simulink model "full_maneuver_platoon_new_strategy"  (R2019a)
settings: Solver=VariableStepAuto  StartTime=0.0  StopTime=70  FixedStep=0.1  MaxStep=0.05  RelTol=1e-3
libraries: simulink x97, dspsigops x7, powerlib_meascontrol x7, autolibshared x7
(part 4 of 7)

== system full_maneuver_platoon_new_strategy/p1/safeErrors ==
  errors : Inport
  AND : Logic  IconShape=distinctive  AllPortsSameDT=off  OutDataTypeStr=boolean
  Compare To Constant4 : simulink/Logic and Bit Operations/Compare To Constant  relop=>=  const=-0.1  OutDataTypeStr=boolean
  Demux : Demux  Outputs=2
  safetyFlag : Outport
  wires:
  Compare To Constant4/1 -> Demux/1
  errors/1 -> Compare To Constant4/1
  AND/1 -> safetyFlag/1
  Demux/1 -> AND/1
  Demux/2 -> AND/2

== system full_maneuver_platoon_new_strategy/p1/safeErrors1 ==
  errors : Inport
  AND : Logic  IconShape=distinctive  AllPortsSameDT=off  OutDataTypeStr=boolean
  Compare To Constant4 : simulink/Logic and Bit Operations/Compare To Constant  relop=>=  const=-0.1  OutDataTypeStr=boolean
  Demux : Demux  Outputs=2
  safetyFlag : Outport
  wires:
  Demux/2 -> AND/2
  Demux/1 -> AND/1
  AND/1 -> safetyFlag/1
  errors/1 -> Compare To Constant4/1
  Compare To Constant4/1 -> Demux/1

== system full_maneuver_platoon_new_strategy/p1/safeErrors2 ==
  errors : Inport
  AND : Logic  IconShape=distinctive  AllPortsSameDT=off  OutDataTypeStr=boolean
  Compare To Constant4 : simulink/Logic and Bit Operations/Compare To Constant  relop=>=  const=-0.1  OutDataTypeStr=boolean
  Demux : Demux  Outputs=2
  safetyFlag : Outport
  wires:
  Compare To Constant4/1 -> Demux/1
  errors/1 -> Compare To Constant4/1
  AND/1 -> safetyFlag/1
  Demux/1 -> AND/1
  Demux/2 -> AND/2

== system full_maneuver_platoon_new_strategy/p1/steadyState ==
  u : Inport
  AND : Logic  IconShape=distinctive  AllPortsSameDT=off  OutDataTypeStr=boolean
  Abs2 : Abs
  Compare To Constant2 : simulink/Logic and Bit Operations/Compare To Constant  relop=<=  const=0.2  OutDataTypeStr=boolean
  Demux : Demux  Outputs=2
  Mux : Mux  Inputs=2
  Transport Delay2 : TransportDelay
  ssFlag : Outport
  wires:
  Demux/2 -> AND/2
  Mux/1 -> Abs2/1
  Compare To Constant2/1 -> Demux/1
  AND/1 -> ssFlag/1
  Transport Delay2/1 -> Mux/1
  Demux/1 -> AND/1
  Abs2/1 -> Compare To Constant2/1
  u/1 -> Mux/2, Transport Delay2/1

== system full_maneuver_platoon_new_strategy/p2/Lateral Control ==
  <Y> : Inport
  <r> : Inport  Port=2
  startLaneChange : Inport  Port=3
  yRef : Inport  Port=4
  Demux2 : Demux
  Full State Observer : Subsystem
  Gain1 : Gain  Gain=Klat  Multiplication=Matrix(K*u)
  Integrator : Integrator  InitialCondition=y0
  Mux : Mux  Inputs=2
  Pad : dspsigops/Pad  padAlong=Columns  dimsToPad=1  valSrc=Specify via dialog  padVal=0  spec=Output size  padNumOutRowsSpecMethod=User-specified  numOutRows=4  padNumOutColsSpecMethod=User-specified  numOutCols=1  isVarDimsMode=off  padBeginning=0  padEnd=0  outSizeMode=User-specified  outSize=1  padSigAt=End  trunc_flag=None  roundingMode=Floor  overflowMode=off  truncOrWrapMode=Truncate  wrap_flag=None
      settings: SourceProductName=DSP System Toolbox  SourceProductBaseCode=DS
  Rate Limiter : RateLimiter  RisingSlewLimit=maxDeltaDot  FallingSlewLimit=-maxDeltaDot  SampleTimeMode=inherited
  Saturation : Saturate  UpperLimit=maxDelta  LowerLimit=-maxDelta
  Scope : Scope  NumInputPorts=4
  Scope1 : Scope
  Sum : Sum  Inputs=|+-
  Sum2 : Sum  Inputs=|+-
  Triggered Subsystem1 : Subsystem  TreatAsAtomicUnit=on
  delta : Outport
  wires:
  Rate Limiter/1 -> Full State Observer/2(delta), Scope1/1, delta/1  "delta"
  Demux2/1 -> Scope/1
  Integrator/1 -> Sum2/2, Pad/1
  Gain1/1 -> Saturation/1
  <r>/1 -> Mux/2
  Full State Observer/1(xhat) -> Sum/2, Demux2/1  "estStates"
  Sum/1 -> Gain1/1
  Pad/1 -> Sum/1
  Mux/1 -> Full State Observer/1(measuredOutputs)
  Demux2/4 -> Scope/4
  Demux2/2 -> Scope/2
  Sum2/1 -> Integrator/1
  Saturation/1 -> Rate Limiter/1
  Demux2/3 -> Scope/3
  Triggered Subsystem1/1(Out1) -> Sum2/1
  <Y>/1 -> Mux/1
  startLaneChange/1 -> Triggered Subsystem1/Trigger
  yRef/1 -> Triggered Subsystem1/1(In1)

== system full_maneuver_platoon_new_strategy/p2/Regular Vehicle Following ==
  ego : Inport
  leader : Inport  Port=2
  extraSpaceFlag : Inport  Port=3
  Bus Selector : BusSelector  OutputSignals=X,Xdot,u
  Bus Selector1 : BusSelector  OutputSignals=X,Xdot
  Chart : Stateflow chart  BlockKeywords=__PRM__SERIALIZED__DATA__:Stateflow Chart,Stateflow Diagram  TreatAsAtomicUnit=on
  Compare To Constant : simulink/Logic and Bit Operations/Compare To Constant  relop=<  const=5*maxHeadwayError  OutDataTypeStr=boolean
  Compare To Constant1 : simulink/Logic and Bit Operations/Compare To Constant  relop=>  const=0  OutDataTypeStr=boolean
  Compute Errors : Subsystem
  Free Flow Velocity Control : Subsystem  TreatAsAtomicUnit=on
  Minimum Velocity Control : Subsystem  TreatAsAtomicUnit=on
  Mux : Mux  Inputs=2
  Rate Limiter : RateLimiter  RisingSlewLimit=maxJerk  FallingSlewLimit=minJerk  SampleTimeMode=inherited
  Rate Limiter1 : RateLimiter  RisingSlewLimit=maxComfJerk  FallingSlewLimit=minComfJerk  SampleTimeMode=inherited
  Scope2 : Scope
  Sum1 : Sum  Inputs=-+|
  Sum6 : Sum  Inputs=-+|
  Switch1 : Switch  Criteria=u2 > Threshold
  Veh Following : Subsystem  TreatAsAtomicUnit=on
  comf saturation : Saturate  UpperLimit=maxComfAccel  LowerLimit=minComfAccel
  freeFlowVel : Constant  Value=freeFlowVel
  output : Scope
  safe saturation : Saturate  UpperLimit=maxAcceleration  LowerLimit=minAcceleration
  vMin : Constant  Value=vMin
  veh foll state : Scope  NumInputPorts=2
  u : Outport
  errors : Outport  Port=2
  gap : Outport  Port=3
  leaderInRange : Outport  Port=4
  wires:
  Bus Selector/2 -> Sum1/1, Sum6/1, Compute Errors/2(vf)  "<Xdot>"
  Bus Selector/1 -> Compute Errors/1(xf)  "<X>"
  extraSpaceFlag/1 -> Compute Errors/5(extraSpaceFlag)
  Compute Errors/1(eh) -> Mux/1, Veh Following/1(eh), Compare To Constant/1
  Compare To Constant/1 -> leaderInRange/1, Chart/1(leaderWithinRange), Free Flow Velocity Control/3(intReset), Veh Following/4(intReset)
  ego/1 -> Bus Selector/1
  Compute Errors/3("gap ") -> gap/1
  Compute Errors/4(unsafeFlag) -> Chart/3(unsafeFlag), Switch1/2, Scope2/1
  Rate Limiter1/1 -> Switch1/3  "sat(u)"
  Bus Selector/3 -> Veh Following/3(realInput), Minimum Velocity Control/2(realInput), Free Flow Velocity Control/2(realInput)  "<u>"
  Chart/2(u) -> safe saturation/1, comf saturation/1, veh foll state/2
  Switch1/1 -> u/1, output/1
  Rate Limiter/1 -> Switch1/1  "sat(u)"
  safe saturation/1 -> Rate Limiter/1
  comf saturation/1 -> Rate Limiter1/1
  Compute Errors/2(ev) -> Veh Following/2(ev), Mux/2
  Free Flow Velocity Control/1(u) -> Chart/5(freeFlowVelControl)
  Bus Selector1/1 -> Compute Errors/3(xl)  "<X>"
  Mux/1 -> errors/1
  Chart/1(state) -> veh foll state/1
  leader/1 -> Bus Selector1/1
  Bus Selector1/2 -> Compute Errors/4(vl)  "<Xdot>"
  Veh Following/1(u) -> Chart/4(vehFoll)  "uVehFoll"
  Sum6/1 -> Compare To Constant1/1, Chart/2(velDiff), Minimum Velocity Control/1(ev)
  Minimum Velocity Control/1(u) -> Chart/6(minVelControl)  "minVelControl"
  vMin/1 -> Sum6/2
  freeFlowVel/1 -> Sum1/2
  Sum1/1 -> Free Flow Velocity Control/1(ev)
  Compare To Constant1/1 -> Minimum Velocity Control/3(intReset)

== system full_maneuver_platoon_new_strategy/p2/Subsystem ==
  note: Condition for Lane Changing Vehicle
  note: Condition for Gap Generating Vehicle
  lcFlag : Inport
  ego : Inport  Port=2  OutDataTypeStr=Bus: vehStatesBus
  virtualLeader : Inport  Port=3  OutDataTypeStr=Bus: vehStatesBus
  lcCanStart : Inport  Port=4
  AND : Logic  IconShape=distinctive  AllPortsSameDT=off  OutDataTypeStr=boolean
  AND1 : Logic  IconShape=distinctive  AllPortsSameDT=off  OutDataTypeStr=boolean
  Abs : Abs
  Bus Selector : BusSelector  OutputSignals=Y
  Bus Selector1 : BusSelector  OutputSignals=Y
  Compare To Constant : simulink/Logic and Bit Operations/Compare To Constant  relop=<  const=3.6-0.5  OutDataTypeStr=boolean
  NOT : Logic  Operator=NOT  IconShape=distinctive  AllPortsSameDT=off  OutDataTypeStr=boolean
  OR : Logic  Operator=OR  IconShape=distinctive  AllPortsSameDT=off  OutDataTypeStr=boolean
  Scope : Scope  NumInputPorts=3
  Sum : Sum  Inputs=+-
  lcStarted : Outport
  wires:
  ego/1 -> Bus Selector/1
  virtualLeader/1 -> Bus Selector1/1
  Bus Selector/1 -> Scope/1, Sum/1  "<Y>"
  Bus Selector1/1 -> Scope/2, Sum/2  "<Y>"
  Compare To Constant/1 -> AND1/1
  Sum/1 -> Abs/1
  Abs/1 -> Scope/3, Compare To Constant/1
  lcFlag/1 -> NOT/1, AND/1
  lcCanStart/1 -> AND/2
  NOT/1 -> AND1/2
  OR/1 -> lcStarted/1
  AND1/1 -> OR/1
  AND/1 -> OR/2

== system full_maneuver_platoon_new_strategy/p2/Subsystem1 ==
  note: Condition for Lane
      | Changing Vehicle
  note: Condition for Gap
      | Generating Vehicle
  ego : Inport  OutDataTypeStr=Bus: vehStatesBus
  futureLeader : Inport  Port=2  OutDataTypeStr=Bus: vehStatesBus
  lcFlag : Inport  Port=3
  AND : Logic  IconShape=distinctive  AllPortsSameDT=off  OutDataTypeStr=boolean
  AND1 : Logic  IconShape=distinctive  AllPortsSameDT=off  OutDataTypeStr=boolean
  Abs : Abs
  Bus Selector1 : BusSelector  OutputSignals=Y
  Bus Selector2 : BusSelector  OutputSignals=Y
  Compare To Constant : simulink/Logic and Bit Operations/Compare To Constant  relop=<=  const=1.8  OutDataTypeStr=boolean
  Compare To Constant1 : simulink/Logic and Bit Operations/Compare To Constant  relop=<=  const=0.5  OutDataTypeStr=boolean
  NOT : Logic  Operator=NOT  IconShape=distinctive  AllPortsSameDT=off  OutDataTypeStr=boolean
  OR : Logic  Operator=OR  IconShape=distinctive  AllPortsSameDT=off  OutDataTypeStr=boolean
  Scope : Scope  NumInputPorts=2
  Sum1 : Sum  Inputs=|+-
  lcDone : Outport
  wires:
  futureLeader/1 -> Bus Selector1/1
  Bus Selector1/1 -> Sum1/2  "<Y>"
  AND/1 -> Scope/1, OR/1
  Compare To Constant/1 -> AND/1
  lcFlag/1 -> AND1/2, NOT/1
  ego/1 -> Bus Selector2/1
  Sum1/1 -> Abs/1
  Compare To Constant1/1 -> AND1/1
  OR/1 -> lcDone/1
  AND1/1 -> Scope/2, OR/2
  Bus Selector2/1 -> Sum1/1  "<Y>"
  Abs/1 -> Compare To Constant1/1, Compare To Constant/1
  NOT/1 -> AND/2

== system full_maneuver_platoon_new_strategy/p2/Triggered Subsystem ==
  Trigger : TriggerPort  VariantControl=Variant
  Constant : Constant
  Out1 : Outport  InitialOutput=0
  wires:
  Constant/1 -> Out1/1

== system full_maneuver_platoon_new_strategy/p2/Triggered Subsystem1 ==
  Trigger : TriggerPort  VariantControl=Variant
  Constant : Constant
  Out1 : Outport  InitialOutput=0
  wires:
  Constant/1 -> Out1/1

== system full_maneuver_platoon_new_strategy/p2/Vehicle Following During LC ==
  ego : Inport
  futureLeader : Inport  Port=2
  extraSpaceFlag : Inport  Port=3
  Enable : EnablePort
  Bus Selector : BusSelector  OutputSignals=X,Xdot,u
  Bus Selector1 : BusSelector  OutputSignals=X,Xdot
  Chart : Stateflow chart  BlockKeywords=__PRM__SERIALIZED__DATA__:Stateflow Chart,Stateflow Diagram  TreatAsAtomicUnit=on
  Compare To Constant : simulink/Logic and Bit Operations/Compare To Constant  relop=<  const=5*maxHeadwayError  OutDataTypeStr=boolean
  Compute Errors : Subsystem
  Mux : Mux  Inputs=2
  Scope : Scope
  Scope3 : Scope
  Terminator : Terminator
  Veh Following : Subsystem  TreatAsAtomicUnit=on
  Velocity Control : Subsystem  TreatAsAtomicUnit=on
  safe acceleration : Saturate  UpperLimit=maxAcceleration  LowerLimit=minAcceleration
  safe jerk : RateLimiter  RisingSlewLimit=maxJerk  FallingSlewLimit=minJerk  SampleTimeMode=inherited
  veh foll state : Scope
  u : Outport  InitialOutput=0
  errors : Outport  Port=2
  gap : Outport  Port=3
  wires:
  futureLeader/1 -> Bus Selector1/1
  Bus Selector/2 -> Velocity Control/1(velocity), Compute Errors/2(vf)  "<Xdot>"
  Compute Errors/1(eh) -> Mux/1, Veh Following/1(eh), Scope/1, Compare To Constant/1
  Compute Errors/4(unsafeFlag) -> Terminator/1
  Chart/1(state) -> veh foll state/1
  Compute Errors/2(ev) -> Veh Following/2(ev), Mux/2
  Bus Selector1/1 -> Compute Errors/3(xl)  "<X>"
  Mux/1 -> errors/1
  extraSpaceFlag/1 -> Compute Errors/5(extraSpaceFlag)
  Bus Selector/3 -> Velocity Control/2(realInput), Veh Following/3(realInput)  "<u>"
  safe jerk/1 -> Scope3/1, u/1  "sat(u)"
  safe acceleration/1 -> safe jerk/1
  Chart/2(u) -> safe acceleration/1
  Velocity Control/1(u) -> Chart/3(uVelControl)
  ego/1 -> Bus Selector/1
  Veh Following/1(u) -> Chart/2(uVehFoll)
  Compare To Constant/1 -> Velocity Control/3(intReset), Veh Following/4(intReset), Chart/1(leaderWithinRange)
  Bus Selector/1 -> Compute Errors/1(xf)  "<X>"
  Compute Errors/3("gap ") -> gap/1
  Bus Selector1/2 -> Compute Errors/4(vl)  "<Xdot>"

== system full_maneuver_platoon_new_strategy/p2/Virtual Vehicle Following ==
  ego : Inport
  virtualLeader : Inport  Port=2
  extraSpaceFlag : Inport  Port=3
  Enable : EnablePort
  Bus Selector : BusSelector  OutputSignals=X,Xdot,u
  Bus Selector1 : BusSelector  OutputSignals=X,Xdot
  Chart : Stateflow chart  BlockKeywords=__PRM__SERIALIZED__DATA__:Stateflow Chart,Stateflow Diagram  TreatAsAtomicUnit=on
  Compute Errors : Subsystem
  Mux : Mux  Inputs=2
  Scope : Scope
  Sum6 : Sum  Inputs=|+-
  Terminator : Terminator
  Transport Delay1 : TransportDelay  DelayTime=0.01
  Velocity Control : Subsystem  TreatAsAtomicUnit=on
  Virtual Leader Following : Subsystem  TreatAsAtomicUnit=on
  accel saturation : Saturate  UpperLimit=maxComfAccel  LowerLimit=minComfAccel
  jerk saturation : RateLimiter  RisingSlewLimit=maxComfJerk  FallingSlewLimit=minComfJerk  SampleTimeMode=inherited
  vMin : Constant  Value=vMin
  u : Outport  InitialOutput=0
  virtualErrors : Outport  Port=2  OutputWhenDisabled=reset  InitialOutput=[0, 0]
  virtualGap : Outport  Port=3  OutputWhenDisabled=reset  InitialOutput=[0]
  wires:
  Sum6/1 -> Velocity Control/2(ev), Chart/1(velDiff)
  virtualLeader/1 -> Bus Selector1/1
  jerk saturation/1 -> Scope/1, u/1  "virtualFoll"
  Mux/1 -> virtualErrors/1
  vMin/1 -> Sum6/1
  Compute Errors/1(eh) -> Virtual Leader Following/1(eh), Mux/1  "eh"
  Bus Selector/3 -> Virtual Leader Following/3(realInput)  "<u>"
  ego/1 -> Bus Selector/1
  Transport Delay1/1 -> Velocity Control/1(intReset)
  Virtual Leader Following/1(u) -> Chart/3(uVehFoll)  "uVehFoll"
  Bus Selector/2 -> Compute Errors/2(vf), Sum6/2  "<Xdot>"
  accel saturation/1 -> jerk saturation/1
  Bus Selector/1 -> Compute Errors/1(xf)  "<X>"
  Compute Errors/3("gap ") -> virtualGap/1
  Chart/2(u) -> accel saturation/1
  Compute Errors/4(unsafeFlag) -> Terminator/1
  Chart/1(state) -> Transport Delay1/1
  Bus Selector1/1 -> Compute Errors/3(xl)  "<X>"
  Velocity Control/1(Out1) -> Chart/2(uVelControl)  "uVelControl"
  Compute Errors/2(ev) -> Mux/2, Virtual Leader Following/2(ev)
  extraSpaceFlag/1 -> Compute Errors/5(lcFlag)
  Bus Selector1/2 -> Compute Errors/4(vl)  "<Xdot>"

== system full_maneuver_platoon_new_strategy/p2/followerErrors ==
  ego : Inport
  follower : Inport  Port=2
  Bus Selector1 : BusSelector  OutputSignals=X,Xdot
  Bus Selector3 : BusSelector  OutputSignals=X,Xdot
  Mux : Mux  Inputs=2
  Sum3 : Sum  Inputs=-+|
  Terminator1 : Terminator
  gapToFollower : Subsystem
  errors : Outport
  wires:
  gapToFollower/2("gap ") -> Terminator1/1
  Sum3/1 -> Mux/2
  Bus Selector3/2 -> gapToFollower/2(vf), Sum3/1  "<Xdot>"
  follower/1 -> Bus Selector3/1
  gapToFollower/1(eh) -> Mux/1
  Bus Selector1/2 -> Sum3/2  "<Xdot>"
  Bus Selector3/1 -> gapToFollower/1(xf)  "<X>"
  ego/1 -> Bus Selector1/1
  Bus Selector1/1 -> gapToFollower/3(xl)  "<X>"
  Mux/1 -> errors/1

== system full_maneuver_platoon_new_strategy/p2/safeErrors ==
  errors : Inport
  AND : Logic  IconShape=distinctive  AllPortsSameDT=off  OutDataTypeStr=boolean
  Compare To Constant4 : simulink/Logic and Bit Operations/Compare To Constant  relop=>=  const=-0.1  OutDataTypeStr=boolean
  Demux : Demux  Outputs=2
  safetyFlag : Outport
  wires:
  Demux/2 -> AND/2
  Demux/1 -> AND/1
  AND/1 -> safetyFlag/1
  errors/1 -> Compare To Constant4/1
  Compare To Constant4/1 -> Demux/1

== system full_maneuver_platoon_new_strategy/p2/safeErrors1 ==
  errors : Inport
  AND : Logic  IconShape=distinctive  AllPortsSameDT=off  OutDataTypeStr=boolean
  Compare To Constant4 : simulink/Logic and Bit Operations/Compare To Constant  relop=>=  const=-0.1  OutDataTypeStr=boolean
  Demux : Demux  Outputs=2
  safetyFlag : Outport
  wires:
  Compare To Constant4/1 -> Demux/1
  errors/1 -> Compare To Constant4/1
  AND/1 -> safetyFlag/1
  Demux/1 -> AND/1
  Demux/2 -> AND/2

== system full_maneuver_platoon_new_strategy/p2/safeErrors2 ==
  errors : Inport
  AND : Logic  IconShape=distinctive  AllPortsSameDT=off  OutDataTypeStr=boolean
  Compare To Constant4 : simulink/Logic and Bit Operations/Compare To Constant  relop=>=  const=-0.1  OutDataTypeStr=boolean
  Demux : Demux  Outputs=2
  safetyFlag : Outport
  wires:
  Demux/2 -> AND/2
  Demux/1 -> AND/1
  AND/1 -> safetyFlag/1
  errors/1 -> Compare To Constant4/1
  Compare To Constant4/1 -> Demux/1

== system full_maneuver_platoon_new_strategy/p2/steadyState ==
  u : Inport
  AND : Logic  IconShape=distinctive  AllPortsSameDT=off  OutDataTypeStr=boolean
  Abs2 : Abs
  Compare To Constant2 : simulink/Logic and Bit Operations/Compare To Constant  relop=<=  const=0.2  OutDataTypeStr=boolean
  Demux : Demux  Outputs=2
  Mux : Mux  Inputs=2
  Transport Delay2 : TransportDelay
  ssFlag : Outport
  wires:
  u/1 -> Transport Delay2/1, Mux/2
  Abs2/1 -> Compare To Constant2/1
  Demux/1 -> AND/1
  Transport Delay2/1 -> Mux/1
  AND/1 -> ssFlag/1
  Compare To Constant2/1 -> Demux/1
  Mux/1 -> Abs2/1
  Demux/2 -> AND/2

== system full_maneuver_platoon_new_strategy/p3/Lateral Control ==
  <Y> : Inport
  <r> : Inport  Port=2
  startLaneChange : Inport  Port=3
  yRef : Inport  Port=4
  Demux2 : Demux
  Full State Observer : Subsystem
  Gain1 : Gain  Gain=Klat  Multiplication=Matrix(K*u)
  Integrator : Integrator  InitialCondition=y0
  Mux : Mux  Inputs=2
  Pad : dspsigops/Pad  padAlong=Columns  dimsToPad=1  valSrc=Specify via dialog  padVal=0  spec=Output size  padNumOutRowsSpecMethod=User-specified  numOutRows=4  padNumOutColsSpecMethod=User-specified  numOutCols=1  isVarDimsMode=off  padBeginning=0  padEnd=0  outSizeMode=User-specified  outSize=1  padSigAt=End  trunc_flag=None  roundingMode=Floor  overflowMode=off  truncOrWrapMode=Truncate  wrap_flag=None
      settings: SourceProductName=DSP System Toolbox  SourceProductBaseCode=DS
  Rate Limiter : RateLimiter  RisingSlewLimit=maxDeltaDot  FallingSlewLimit=-maxDeltaDot  SampleTimeMode=inherited
  Saturation : Saturate  UpperLimit=maxDelta  LowerLimit=-maxDelta
  Scope : Scope  NumInputPorts=4
  Scope1 : Scope
  Sum : Sum  Inputs=|+-
  Sum2 : Sum  Inputs=|+-
  Triggered Subsystem1 : Subsystem  TreatAsAtomicUnit=on
  delta : Outport
  wires:
  yRef/1 -> Triggered Subsystem1/1(In1)
  startLaneChange/1 -> Triggered Subsystem1/Trigger
  <Y>/1 -> Mux/1
  Triggered Subsystem1/1(Out1) -> Sum2/1
  Demux2/3 -> Scope/3
  Saturation/1 -> Rate Limiter/1
  Sum2/1 -> Integrator/1
  Demux2/2 -> Scope/2
  Demux2/4 -> Scope/4
  Mux/1 -> Full State Observer/1(measuredOutputs)
  Pad/1 -> Sum/1
  Sum/1 -> Gain1/1
  Full State Observer/1(xhat) -> Demux2/1, Sum/2  "estStates"
  <r>/1 -> Mux/2
  Gain1/1 -> Saturation/1
  Integrator/1 -> Pad/1, Sum2/2
  Demux2/1 -> Scope/1
  Rate Limiter/1 -> delta/1, Scope1/1, Full State Observer/2(delta)  "delta"

== system full_maneuver_platoon_new_strategy/p3/Regular Vehicle Following ==
  ego : Inport
  leader : Inport  Port=2
  extraSpaceFlag : Inport  Port=3
  Bus Selector : BusSelector  OutputSignals=X,Xdot,u
  Bus Selector1 : BusSelector  OutputSignals=X,Xdot
  Chart : Stateflow chart  BlockKeywords=__PRM__SERIALIZED__DATA__:Stateflow Chart,Stateflow Diagram  TreatAsAtomicUnit=on
  Compare To Constant : simulink/Logic and Bit Operations/Compare To Constant  relop=<  const=5*maxHeadwayError  OutDataTypeStr=boolean
  Compare To Constant1 : simulink/Logic and Bit Operations/Compare To Constant  relop=>  const=0  OutDataTypeStr=boolean
  Compute Errors : Subsystem
  Free Flow Velocity Control : Subsystem  TreatAsAtomicUnit=on
  Minimum Velocity Control : Subsystem  TreatAsAtomicUnit=on
  Mux : Mux  Inputs=2
  Rate Limiter : RateLimiter  RisingSlewLimit=maxJerk  FallingSlewLimit=minJerk  SampleTimeMode=inherited
  Rate Limiter1 : RateLimiter  RisingSlewLimit=maxComfJerk  FallingSlewLimit=minComfJerk  SampleTimeMode=inherited
  Scope2 : Scope
  Sum1 : Sum  Inputs=-+|
  Sum6 : Sum  Inputs=-+|
  Switch1 : Switch  Criteria=u2 > Threshold
  Veh Following : Subsystem  TreatAsAtomicUnit=on
  comf saturation : Saturate  UpperLimit=maxComfAccel  LowerLimit=minComfAccel
  freeFlowVel : Constant  Value=freeFlowVel
  output : Scope
  safe saturation : Saturate  UpperLimit=maxAcceleration  LowerLimit=minAcceleration
  vMin : Constant  Value=vMin
  veh foll state : Scope  NumInputPorts=2
  u : Outport
  errors : Outport  Port=2
  gap : Outport  Port=3
  leaderInRange : Outport  Port=4
  wires:
  Compare To Constant1/1 -> Minimum Velocity Control/3(intReset)
  Sum1/1 -> Free Flow Velocity Control/1(ev)
  freeFlowVel/1 -> Sum1/2
  vMin/1 -> Sum6/2
  Minimum Velocity Control/1(u) -> Chart/6(minVelControl)  "minVelControl"
  Sum6/1 -> Minimum Velocity Control/1(ev), Chart/2(velDiff), Compare To Constant1/1
  Veh Following/1(u) -> Chart/4(vehFoll)  "uVehFoll"
  Bus Selector1/2 -> Compute Errors/4(vl)  "<Xdot>"
  leader/1 -> Bus Selector1/1
  Chart/1(state) -> veh foll state/1
  Mux/1 -> errors/1
  Bus Selector1/1 -> Compute Errors/3(xl)  "<X>"
  Free Flow Velocity Control/1(u) -> Chart/5(freeFlowVelControl)
  Compute Errors/2(ev) -> Mux/2, Veh Following/2(ev)
  comf saturation/1 -> Rate Limiter1/1
  safe saturation/1 -> Rate Limiter/1
  Rate Limiter/1 -> Switch1/1  "sat(u)"
  Switch1/1 -> output/1, u/1
  Chart/2(u) -> veh foll state/2, comf saturation/1, safe saturation/1
  Bus Selector/3 -> Free Flow Velocity Control/2(realInput), Minimum Velocity Control/2(realInput), Veh Following/3(realInput)  "<u>"
  Rate Limiter1/1 -> Switch1/3  "sat(u)"
  Compute Errors/4(unsafeFlag) -> Scope2/1, Switch1/2, Chart/3(unsafeFlag)
  Compute Errors/3("gap ") -> gap/1
  ego/1 -> Bus Selector/1
  Compare To Constant/1 -> Veh Following/4(intReset), Free Flow Velocity Control/3(intReset), Chart/1(leaderWithinRange), leaderInRange/1
  Compute Errors/1(eh) -> Compare To Constant/1, Veh Following/1(eh), Mux/1
  extraSpaceFlag/1 -> Compute Errors/5(extraSpaceFlag)
  Bus Selector/1 -> Compute Errors/1(xf)  "<X>"
  Bus Selector/2 -> Compute Errors/2(vf), Sum6/1, Sum1/1  "<Xdot>"

== system full_maneuver_platoon_new_strategy/p3/Subsystem ==
  note: Condition for Gap Generating Vehicle
  note: Condition for Lane Changing Vehicle
  lcFlag : Inport
  ego : Inport  Port=2  OutDataTypeStr=Bus: vehStatesBus
  virtualLeader : Inport  Port=3  OutDataTypeStr=Bus: vehStatesBus
  lcCanStart : Inport  Port=4
  AND : Logic  IconShape=distinctive  AllPortsSameDT=off  OutDataTypeStr=boolean
  AND1 : Logic  IconShape=distinctive  AllPortsSameDT=off  OutDataTypeStr=boolean
  Abs : Abs
  Bus Selector : BusSelector  OutputSignals=Y
  Bus Selector1 : BusSelector  OutputSignals=Y
  Compare To Constant : simulink/Logic and Bit Operations/Compare To Constant  relop=<  const=3.6-0.5  OutDataTypeStr=boolean
  NOT : Logic  Operator=NOT  IconShape=distinctive  AllPortsSameDT=off  OutDataTypeStr=boolean
  OR : Logic  Operator=OR  IconShape=distinctive  AllPortsSameDT=off  OutDataTypeStr=boolean
  Scope : Scope  NumInputPorts=3
  Sum : Sum  Inputs=+-
  lcStarted : Outport
  wires:
  AND/1 -> OR/2
  AND1/1 -> OR/1
  OR/1 -> lcStarted/1
  NOT/1 -> AND1/2
  lcCanStart/1 -> AND/2
  lcFlag/1 -> AND/1, NOT/1
  Abs/1 -> Compare To Constant/1, Scope/3
  Sum/1 -> Abs/1
  Compare To Constant/1 -> AND1/1
  Bus Selector1/1 -> Sum/2, Scope/2  "<Y>"
  Bus Selector/1 -> Sum/1, Scope/1  "<Y>"
  virtualLeader/1 -> Bus Selector1/1
  ego/1 -> Bus Selector/1

== system full_maneuver_platoon_new_strategy/p3/Subsystem1 ==
  note: Condition for Gap
      | Generating Vehicle
  note: Condition for Lane
      | Changing Vehicle
  ego : Inport  OutDataTypeStr=Bus: vehStatesBus
  futureLeader : Inport  Port=2  OutDataTypeStr=Bus: vehStatesBus
  lcFlag : Inport  Port=3
  AND : Logic  IconShape=distinctive  AllPortsSameDT=off  OutDataTypeStr=boolean
  AND1 : Logic  IconShape=distinctive  AllPortsSameDT=off  OutDataTypeStr=boolean
  Abs : Abs
  Bus Selector1 : BusSelector  OutputSignals=Y
  Bus Selector2 : BusSelector  OutputSignals=Y
  Compare To Constant : simulink/Logic and Bit Operations/Compare To Constant  relop=<=  const=1.8  OutDataTypeStr=boolean
  Compare To Constant1 : simulink/Logic and Bit Operations/Compare To Constant  relop=<=  const=0.5  OutDataTypeStr=boolean
  NOT : Logic  Operator=NOT  IconShape=distinctive  AllPortsSameDT=off  OutDataTypeStr=boolean
  OR : Logic  Operator=OR  IconShape=distinctive  AllPortsSameDT=off  OutDataTypeStr=boolean
  Scope : Scope  NumInputPorts=2
  Sum1 : Sum  Inputs=|+-
  lcDone : Outport
  wires:
  NOT/1 -> AND/2
  Abs/1 -> Compare To Constant/1, Compare To Constant1/1
  Bus Selector2/1 -> Sum1/1  "<Y>"
  AND1/1 -> OR/2, Scope/2
  OR/1 -> lcDone/1
  Compare To Constant1/1 -> AND1/1
  Sum1/1 -> Abs/1
  ego/1 -> Bus Selector2/1
  lcFlag/1 -> NOT/1, AND1/2
  Compare To Constant/1 -> AND/1
  AND/1 -> OR/1, Scope/1
  Bus Selector1/1 -> Sum1/2  "<Y>"
  futureLeader/1 -> Bus Selector1/1

== system full_maneuver_platoon_new_strategy/p3/Triggered Subsystem ==
  Trigger : TriggerPort  VariantControl=Variant
  Constant : Constant
  Out1 : Outport  InitialOutput=0
  wires:
  Constant/1 -> Out1/1

== system full_maneuver_platoon_new_strategy/p3/Triggered Subsystem1 ==
  Trigger : TriggerPort  VariantControl=Variant
  Constant : Constant
  Out1 : Outport  InitialOutput=0
  wires:
  Constant/1 -> Out1/1

== system full_maneuver_platoon_new_strategy/p3/Vehicle Following During LC ==
  ego : Inport
  futureLeader : Inport  Port=2
  extraSpaceFlag : Inport  Port=3
  Enable : EnablePort
  Bus Selector : BusSelector  OutputSignals=X,Xdot,u
  Bus Selector1 : BusSelector  OutputSignals=X,Xdot
  Chart : Stateflow chart  BlockKeywords=__PRM__SERIALIZED__DATA__:Stateflow Chart,Stateflow Diagram  TreatAsAtomicUnit=on
  Compare To Constant : simulink/Logic and Bit Operations/Compare To Constant  relop=<  const=5*maxHeadwayError  OutDataTypeStr=boolean
  Compute Errors : Subsystem
  Mux : Mux  Inputs=2
  Scope : Scope
  Scope3 : Scope
  Terminator : Terminator
  Veh Following : Subsystem  TreatAsAtomicUnit=on
  Velocity Control : Subsystem  TreatAsAtomicUnit=on
  safe acceleration : Saturate  UpperLimit=maxAcceleration  LowerLimit=minAcceleration
  safe jerk : RateLimiter  RisingSlewLimit=maxJerk  FallingSlewLimit=minJerk  SampleTimeMode=inherited
  veh foll state : Scope
  u : Outport  InitialOutput=0
  errors : Outport  Port=2
  gap : Outport  Port=3
  wires:
  Bus Selector1/2 -> Compute Errors/4(vl)  "<Xdot>"
  Compute Errors/3("gap ") -> gap/1
  Bus Selector/1 -> Compute Errors/1(xf)  "<X>"
  Compare To Constant/1 -> Chart/1(leaderWithinRange), Veh Following/4(intReset), Velocity Control/3(intReset)
  Veh Following/1(u) -> Chart/2(uVehFoll)
  ego/1 -> Bus Selector/1
  Velocity Control/1(u) -> Chart/3(uVelControl)
  Chart/2(u) -> safe acceleration/1
  safe acceleration/1 -> safe jerk/1
  safe jerk/1 -> u/1, Scope3/1  "sat(u)"
  Bus Selector/3 -> Veh Following/3(realInput), Velocity Control/2(realInput)  "<u>"
  extraSpaceFlag/1 -> Compute Errors/5(extraSpaceFlag)
  Mux/1 -> errors/1
  Bus Selector1/1 -> Compute Errors/3(xl)  "<X>"
  Compute Errors/2(ev) -> Mux/2, Veh Following/2(ev)
  Chart/1(state) -> veh foll state/1
  Compute Errors/4(unsafeFlag) -> Terminator/1
  Compute Errors/1(eh) -> Compare To Constant/1, Scope/1, Veh Following/1(eh), Mux/1
  Bus Selector/2 -> Compute Errors/2(vf), Velocity Control/1(velocity)  "<Xdot>"
  futureLeader/1 -> Bus Selector1/1

== system full_maneuver_platoon_new_strategy/p3/Virtual Vehicle Following ==
  ego : Inport
  virtualLeader : Inport  Port=2
  extraSpaceFlag : Inport  Port=3
  Enable : EnablePort
  Bus Selector : BusSelector  OutputSignals=X,Xdot,u
  Bus Selector1 : BusSelector  OutputSignals=X,Xdot
  Chart : Stateflow chart  BlockKeywords=__PRM__SERIALIZED__DATA__:Stateflow Chart,Stateflow Diagram  TreatAsAtomicUnit=on
  Compute Errors : Subsystem
  Mux : Mux  Inputs=2
  Scope : Scope
  Sum6 : Sum  Inputs=|+-
  Terminator : Terminator
  Transport Delay1 : TransportDelay  DelayTime=0.01
  Velocity Control : Subsystem  TreatAsAtomicUnit=on
  Virtual Leader Following : Subsystem  TreatAsAtomicUnit=on
  accel saturation : Saturate  UpperLimit=maxComfAccel  LowerLimit=minComfAccel
  jerk saturation : RateLimiter  RisingSlewLimit=maxComfJerk  FallingSlewLimit=minComfJerk  SampleTimeMode=inherited
  vMin : Constant  Value=vMin
  u : Outport  InitialOutput=0
  virtualErrors : Outport  Port=2  OutputWhenDisabled=reset  InitialOutput=[0, 0]
  virtualGap : Outport  Port=3  OutputWhenDisabled=reset  InitialOutput=[0]
  wires:
  Bus Selector1/2 -> Compute Errors/4(vl)  "<Xdot>"
  extraSpaceFlag/1 -> Compute Errors/5(lcFlag)
  Compute Errors/2(ev) -> Virtual Leader Following/2(ev), Mux/2
  Velocity Control/1(Out1) -> Chart/2(uVelControl)  "uVelControl"
  Bus Selector1/1 -> Compute Errors/3(xl)  "<X>"
  Chart/1(state) -> Transport Delay1/1
  Compute Errors/4(unsafeFlag) -> Terminator/1
  Chart/2(u) -> accel saturation/1
  Compute Errors/3("gap ") -> virtualGap/1
  Bus Selector/1 -> Compute Errors/1(xf)  "<X>"
  accel saturation/1 -> jerk saturation/1
  Bus Selector/2 -> Sum6/2, Compute Errors/2(vf)  "<Xdot>"
  Virtual Leader Following/1(u) -> Chart/3(uVehFoll)  "uVehFoll"
  Transport Delay1/1 -> Velocity Control/1(intReset)
  ego/1 -> Bus Selector/1
  Bus Selector/3 -> Virtual Leader Following/3(realInput)  "<u>"
  Compute Errors/1(eh) -> Mux/1, Virtual Leader Following/1(eh)  "eh"
  vMin/1 -> Sum6/1
  Mux/1 -> virtualErrors/1
  jerk saturation/1 -> u/1, Scope/1  "virtualFoll"
  virtualLeader/1 -> Bus Selector1/1
  Sum6/1 -> Chart/1(velDiff), Velocity Control/2(ev)

== system full_maneuver_platoon_new_strategy/p3/followerErrors ==
  ego : Inport
  follower : Inport  Port=2
  Bus Selector1 : BusSelector  OutputSignals=X,Xdot
  Bus Selector3 : BusSelector  OutputSignals=X,Xdot
  Mux : Mux  Inputs=2
  Sum3 : Sum  Inputs=-+|
  Terminator1 : Terminator
  gapToFollower : Subsystem
  errors : Outport
  wires:
  Mux/1 -> errors/1
  Bus Selector1/1 -> gapToFollower/3(xl)  "<X>"
  ego/1 -> Bus Selector1/1
  Bus Selector3/1 -> gapToFollower/1(xf)  "<X>"
  Bus Selector1/2 -> Sum3/2  "<Xdot>"
  gapToFollower/1(eh) -> Mux/1
  follower/1 -> Bus Selector3/1
  Bus Selector3/2 -> Sum3/1, gapToFollower/2(vf)  "<Xdot>"
  Sum3/1 -> Mux/2
  gapToFollower/2("gap ") -> Terminator1/1

== system full_maneuver_platoon_new_strategy/p3/safeErrors ==
  errors : Inport
  AND : Logic  IconShape=distinctive  AllPortsSameDT=off  OutDataTypeStr=boolean
  Compare To Constant4 : simulink/Logic and Bit Operations/Compare To Constant  relop=>=  const=-0.1  OutDataTypeStr=boolean
  Demux : Demux  Outputs=2
  safetyFlag : Outport
  wires:
  Compare To Constant4/1 -> Demux/1
  errors/1 -> Compare To Constant4/1
  AND/1 -> safetyFlag/1
  Demux/1 -> AND/1
  Demux/2 -> AND/2

== system full_maneuver_platoon_new_strategy/p3/safeErrors1 ==
  errors : Inport
  AND : Logic  IconShape=distinctive  AllPortsSameDT=off  OutDataTypeStr=boolean
  Compare To Constant4 : simulink/Logic and Bit Operations/Compare To Constant  relop=>=  const=-0.1  OutDataTypeStr=boolean
  Demux : Demux  Outputs=2
  safetyFlag : Outport
  wires:
  Demux/2 -> AND/2
  Demux/1 -> AND/1
  AND/1 -> safetyFlag/1
  errors/1 -> Compare To Constant4/1
  Compare To Constant4/1 -> Demux/1

== system full_maneuver_platoon_new_strategy/p3/safeErrors2 ==
  errors : Inport
  AND : Logic  IconShape=distinctive  AllPortsSameDT=off  OutDataTypeStr=boolean
  Compare To Constant4 : simulink/Logic and Bit Operations/Compare To Constant  relop=>=  const=-0.1  OutDataTypeStr=boolean
  Demux : Demux  Outputs=2
  safetyFlag : Outport
  wires:
  Compare To Constant4/1 -> Demux/1
  errors/1 -> Compare To Constant4/1
  AND/1 -> safetyFlag/1
  Demux/1 -> AND/1
  Demux/2 -> AND/2

== system full_maneuver_platoon_new_strategy/p3/steadyState ==
  u : Inport
  AND : Logic  IconShape=distinctive  AllPortsSameDT=off  OutDataTypeStr=boolean
  Abs2 : Abs
  Compare To Constant2 : simulink/Logic and Bit Operations/Compare To Constant  relop=<=  const=0.2  OutDataTypeStr=boolean
  Demux : Demux  Outputs=2
  Mux : Mux  Inputs=2
  Transport Delay2 : TransportDelay
  ssFlag : Outport
  wires:
  Demux/2 -> AND/2
  Mux/1 -> Abs2/1
  Compare To Constant2/1 -> Demux/1
  AND/1 -> ssFlag/1
  Transport Delay2/1 -> Mux/1
  Demux/1 -> AND/1
  Abs2/1 -> Compare To Constant2/1
  u/1 -> Mux/2, Transport Delay2/1

== system full_maneuver_platoon_new_strategy/Fd/Lateral Control/Full State Observer ==
  note: yhat
  note: xhat
  measuredOutputs : Inport
  delta : Inport  Port=2
  Add1 : Sum  Inputs=|-+
  Gain : Gain  Gain=B  Multiplication=Matrix(K*u)
  Gain1 : Gain  Gain=C  Multiplication=Matrix(K*u)
  Gain2 : Gain  Gain=L  Multiplication=Matrix(K*u)
  Gain3 : Gain  Gain=A  Multiplication=Matrix(K*u)
  Integrator : Integrator  InitialCondition=[y0; 0; 0; 0]
  Signal Specification : SignalSpecification  Dimensions=[size(C,1) 1]
  Sum : Sum  Inputs=+++
  xhat : Outport
  wires:
  Gain2/1 -> Sum/1
  Signal Specification/1 -> Gain2/1
  Gain3/1 -> Sum/2
  Gain/1 -> Sum/3
  delta/1 -> Gain/1
  measuredOutputs/1 -> Add1/2
  Sum/1 -> Integrator/1
  Gain1/1 -> Add1/1
  Integrator/1 -> Gain1/1, Gain3/1, xhat/1
  Add1/1 -> Signal Specification/1

== system full_maneuver_platoon_new_strategy/Fd/Lateral Control/Triggered Subsystem1 ==
  In1 : Inport
  Trigger : TriggerPort  VariantControl=Variant
  Out1 : Outport  InitialOutput=y0
  wires:
  In1/1 -> Out1/1

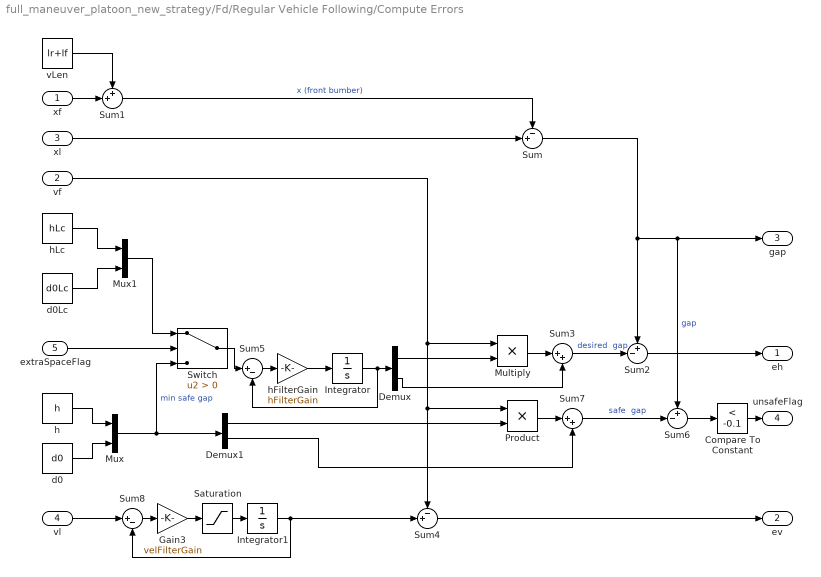
== system full_maneuver_platoon_new_strategy/Fd/Regular Vehicle Following/Compute Errors ==
  xf : Inport
  vf : Inport  Port=2
  xl : Inport  Port=3
  vl : Inport  Port=4
  extraSpaceFlag : Inport  Port=5
  Compare To Constant : simulink/Logic and Bit Operations/Compare To Constant  relop=<  const=-0.1  OutDataTypeStr=boolean
  Demux : Demux  Outputs=2
  Demux1 : Demux  Outputs=2
  Gain3 : Gain  Gain=velFilterGain
  Integrator : Integrator  InitialCondition=[h d0]
  Integrator1 : Integrator  InitialCondition=vx0
  Multiply : Product
  Mux : Mux  Inputs=2
  Mux1 : Mux  Inputs=2
  Product : Product
  Saturation : Saturate  UpperLimit=maxAcceleration  LowerLimit=minAcceleration
  Sum : Sum  Inputs=-+|
  Sum1 : Sum  Inputs=++|
  Sum2 : Sum  Inputs=+-|
  Sum3 : Sum  Inputs=|++
  Sum4 : Sum  Inputs=-+|
  Sum5 : Sum  Inputs=|+-
  Sum6 : Sum  Inputs=+-|
  Sum7 : Sum  Inputs=|++
  Sum8 : Sum  Inputs=|+-
  Switch : Switch  Criteria=u2 > Threshold
  d0 : Constant  Value=d0
  d0Lc : Constant  Value=d0Lc
  h : Constant  Value=h
  hFilterGain : Gain  Gain=hFilterGain
  hLc : Constant  Value=hLc
  vLen : Constant  Value=lr+lf
  eh : Outport
  ev : Outport  Port=2
  "gap " : Outport  Port=3
  unsafeFlag : Outport  Port=4
  wires:
  Sum6/1 -> Compare To Constant/1
  Mux/1 -> Switch/3, Demux1/1  "min safe gap"
  Sum7/1 -> Sum6/2  "safe  gap"
  Mux1/1 -> Switch/1
  d0/1 -> Mux/2
  Integrator/1 -> Demux/1, Sum5/2
  Demux1/1 -> Product/2
  Compare To Constant/1 -> unsafeFlag/1
  Sum2/1 -> eh/1
  extraSpaceFlag/1 -> Switch/2
  xl/1 -> Sum/2
  Product/1 -> Sum7/1
  h/1 -> Mux/1
  Sum3/1 -> Sum2/2  "desired  gap"
  Sum1/1 -> Sum/1  "x (front bumber)"
  vf/1 -> Sum4/1, Product/1, Multiply/1
  Sum5/1 -> hFilterGain/1
  Switch/1 -> Sum5/1
  Demux/2 -> Sum3/2
  vLen/1 -> Sum1/1
  hLc/1 -> Mux1/1
  Demux1/2 -> Sum7/2
  Multiply/1 -> Sum3/1
  Sum/1 -> Sum6/1, "gap "/1, Sum2/1  "gap"
  xf/1 -> Sum1/2
  Demux/1 -> Multiply/2
  hFilterGain/1 -> Integrator/1
  d0Lc/1 -> Mux1/2
  vl/1 -> Sum8/1
  Sum4/1 -> ev/1
  Gain3/1 -> Saturation/1
  Saturation/1 -> Integrator1/1
  Integrator1/1 -> Sum4/2, Sum8/2
  Sum8/1 -> Gain3/1

== system full_maneuver_platoon_new_strategy/Fd/Regular Vehicle Following/Veh Following ==
  eh : Inport
  ev : Inport  Port=2
  realInput : Inport  Port=3
  intReset : Inport  Port=4
  Anti-windup gain : Gain  Gain=sqrt(Ki/Kd)
  Integrator : Integrator  ExternalReset=rising
  Kd : Gain  Gain=Kd
  Ki : Gain  Gain=Ki
  Kp : Gain  Gain=Kp
  Saturation1 : Saturate  UpperLimit=maxHeadwayError  LowerLimit=minHeadwayError
  Scope : Scope  NumInputPorts=4
  Sum : Sum  Inputs=|-+
  Sum1 : Sum  Inputs=+++
  Sum5 : Sum  Inputs=-+|
  u : Outport
  wires:
  ev/1 -> Kd/1
  Ki/1 -> Sum5/2
  Anti-windup gain/1 -> Sum5/1
  Sum5/1 -> Integrator/1
  Integrator/1 -> Sum1/1, Scope/1
  Kp/1 -> Sum1/2, Scope/2
  Kd/1 -> Scope/3, Sum1/3
  Saturation1/1 -> Kp/1, Ki/1
  eh/1 -> Saturation1/1
  Sum1/1 -> Sum/2, u/1, Scope/4
  realInput/1 -> Sum/1
  Sum/1 -> Anti-windup gain/1
  intReset/1 -> Integrator/2

== system full_maneuver_platoon_new_strategy/Fd/Regular Vehicle Following/Velocity Control ==
  velocity : Inport
  realInput : Inport  Port=2
  intReset : Inport  Port=3
  Anti-windup gain : Gain  Gain=velKp/velKi
  Integrator2 : Integrator  ExternalReset=falling
  Sum : Sum  Inputs=|+-
  Sum1 : Sum  Inputs=|-+
  Sum2 : Sum  Inputs=-+|
  Sum3 : Sum  Inputs=|++
  freeFlowVel : Constant  Value=freeFlowVel
  velKi : Gain  Gain=velKi
  velKp : Gain  Gain=velKp
  u : Outport
  wires:
  Sum/1 -> velKi/1, velKp/1
  velKp/1 -> Sum3/2
  velKi/1 -> Sum2/2
  Integrator2/1 -> Sum3/1
  velocity/1 -> Sum/2
  freeFlowVel/1 -> Sum/1
  intReset/1 -> Integrator2/2
  Sum3/1 -> Sum1/2, u/1
  Anti-windup gain/1 -> Sum2/1
  realInput/1 -> Sum1/1
  Sum1/1 -> Anti-windup gain/1
  Sum2/1 -> Integrator2/1

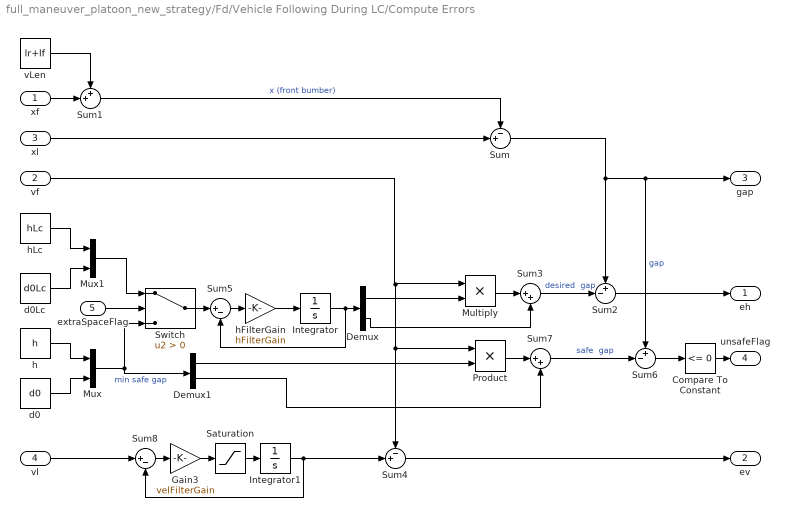
== system full_maneuver_platoon_new_strategy/Fd/Vehicle Following During LC/Compute Errors ==
  xf : Inport
  vf : Inport  Port=2
  xl : Inport  Port=3
  vl : Inport  Port=4
  extraSpaceFlag : Inport  Port=5
  Compare To Constant : simulink/Logic and Bit Operations/Compare To Constant  relop=<=  const=0  OutDataTypeStr=boolean
  Demux : Demux  Outputs=2
  Demux1 : Demux  Outputs=2
  Gain3 : Gain  Gain=velFilterGain
  Integrator : Integrator  InitialCondition=[h d0]
  Integrator1 : Integrator  InitialCondition=vx0
  Multiply : Product
  Mux : Mux  Inputs=2
  Mux1 : Mux  Inputs=2
  Product : Product
  Saturation : Saturate  UpperLimit=maxAcceleration  LowerLimit=minAcceleration
  Sum : Sum  Inputs=-+|
  Sum1 : Sum  Inputs=++|
  Sum2 : Sum  Inputs=+-|
  Sum3 : Sum  Inputs=|++
  Sum4 : Sum  Inputs=-+|
  Sum5 : Sum  Inputs=|+-
  Sum6 : Sum  Inputs=+-|
  Sum7 : Sum  Inputs=|++
  Sum8 : Sum  Inputs=|+-
  Switch : Switch  Criteria=u2 > Threshold
  d0 : Constant  Value=d0
  d0Lc : Constant  Value=d0Lc
  h : Constant  Value=h
  hFilterGain : Gain  Gain=hFilterGain
  hLc : Constant  Value=hLc
  vLen : Constant  Value=lr+lf
  eh : Outport
  ev : Outport  Port=2
  "gap " : Outport  Port=3
  unsafeFlag : Outport  Port=4
  wires:
  Sum4/1 -> ev/1
  d0Lc/1 -> Mux1/2
  hFilterGain/1 -> Integrator/1
  Demux/1 -> Multiply/2
  xf/1 -> Sum1/2
  Sum/1 -> Sum2/1, "gap "/1, Sum6/1  "gap"
  Multiply/1 -> Sum3/1
  Demux1/2 -> Sum7/2
  hLc/1 -> Mux1/1
  vLen/1 -> Sum1/1
  Demux/2 -> Sum3/2
  Switch/1 -> Sum5/1
  Sum5/1 -> hFilterGain/1
  vf/1 -> Multiply/1, Product/1, Sum4/1
  Sum1/1 -> Sum/1  "x (front bumber)"
  Sum3/1 -> Sum2/2  "desired  gap"
  h/1 -> Mux/1
  Product/1 -> Sum7/1
  xl/1 -> Sum/2
  extraSpaceFlag/1 -> Switch/2
  Sum2/1 -> eh/1
  Compare To Constant/1 -> unsafeFlag/1
  Demux1/1 -> Product/2
  Integrator/1 -> Sum5/2, Demux/1
  d0/1 -> Mux/2
  Mux1/1 -> Switch/1
  Sum7/1 -> Sum6/2  "safe  gap"
  Mux/1 -> Switch/3, Demux1/1  "min safe gap"
  Sum6/1 -> Compare To Constant/1
  Saturation/1 -> Integrator1/1
  Gain3/1 -> Saturation/1
  Integrator1/1 -> Sum4/2, Sum8/2
  Sum8/1 -> Gain3/1
  vl/1 -> Sum8/1

== system full_maneuver_platoon_new_strategy/Fd/Vehicle Following During LC/Veh Following ==
  eh : Inport
  ev : Inport  Port=2
  realInput : Inport  Port=3
  intReset : Inport  Port=4
  Anti-windup gain : Gain  Gain=sqrt(Ki/Kd)
  Integrator : Integrator  ExternalReset=rising
  Kd : Gain  Gain=Kd
  Ki : Gain  Gain=Ki
  Kp : Gain  Gain=Kp
  Saturation1 : Saturate  UpperLimit=maxHeadwayError  LowerLimit=minHeadwayError
  Scope : Scope  NumInputPorts=4
  Sum : Sum  Inputs=|-+
  Sum1 : Sum  Inputs=+++
  Sum5 : Sum  Inputs=-+|
  u : Outport
  wires:
  intReset/1 -> Integrator/2
  Sum/1 -> Anti-windup gain/1
  realInput/1 -> Sum/1
  Sum1/1 -> Scope/4, u/1, Sum/2
  eh/1 -> Saturation1/1
  Saturation1/1 -> Ki/1, Kp/1
  Kd/1 -> Sum1/3, Scope/3
  Kp/1 -> Scope/2, Sum1/2
  Integrator/1 -> Scope/1, Sum1/1
  Sum5/1 -> Integrator/1
  Anti-windup gain/1 -> Sum5/1
  Ki/1 -> Sum5/2
  ev/1 -> Kd/1

== system full_maneuver_platoon_new_strategy/Fd/Vehicle Following During LC/Velocity Control ==
  velocity : Inport
  realInput : Inport  Port=2
  intReset : Inport  Port=3
  Anti-windup gain : Gain  Gain=velKp/velKi
  Integrator2 : Integrator  ExternalReset=falling
  Sum : Sum  Inputs=|+-
  Sum1 : Sum  Inputs=|-+
  Sum2 : Sum  Inputs=-+|
  Sum3 : Sum  Inputs=|++
  freeFlowVel : Constant  Value=freeFlowVel
  velKi : Gain  Gain=velKi
  velKp : Gain  Gain=velKp
  u : Outport
  wires:
  Sum2/1 -> Integrator2/1
  Sum1/1 -> Anti-windup gain/1
  realInput/1 -> Sum1/1
  Anti-windup gain/1 -> Sum2/1
  Sum3/1 -> u/1, Sum1/2
  intReset/1 -> Integrator2/2
  freeFlowVel/1 -> Sum/1
  velocity/1 -> Sum/2
  Integrator2/1 -> Sum3/1
  velKi/1 -> Sum2/2
  velKp/1 -> Sum3/2
  Sum/1 -> velKp/1, velKi/1

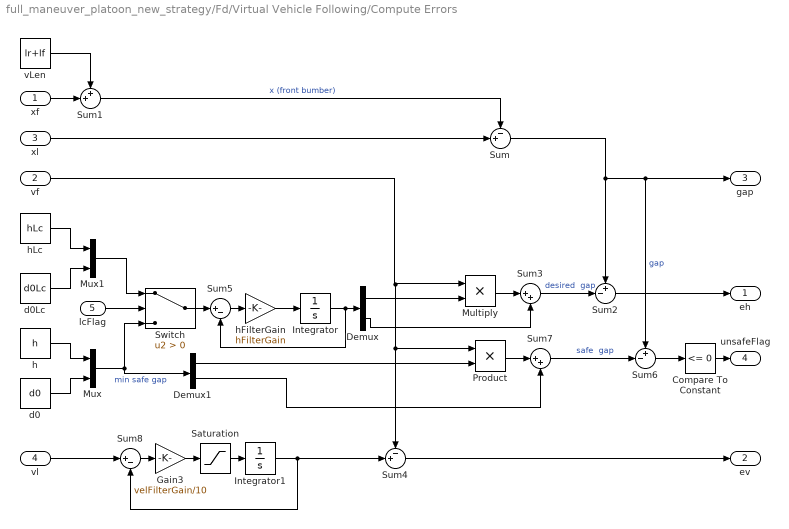
== system full_maneuver_platoon_new_strategy/Fd/Virtual Vehicle Following/Compute Errors ==
  xf : Inport
  vf : Inport  Port=2
  xl : Inport  Port=3
  vl : Inport  Port=4
  lcFlag : Inport  Port=5
  Compare To Constant : simulink/Logic and Bit Operations/Compare To Constant  relop=<=  const=0  OutDataTypeStr=boolean
  Demux : Demux  Outputs=2
  Demux1 : Demux  Outputs=2
  Gain3 : Gain  Gain=velFilterGain/10
  Integrator : Integrator  InitialCondition=[h d0]
  Integrator1 : Integrator  InitialCondition=vx0
  Multiply : Product
  Mux : Mux  Inputs=2
  Mux1 : Mux  Inputs=2
  Product : Product
  Saturation : Saturate  UpperLimit=maxAcceleration  LowerLimit=minAcceleration
  Sum : Sum  Inputs=-+|
  Sum1 : Sum  Inputs=++|
  Sum2 : Sum  Inputs=+-|
  Sum3 : Sum  Inputs=|++
  Sum4 : Sum  Inputs=-+|
  Sum5 : Sum  Inputs=|+-
  Sum6 : Sum  Inputs=+-|
  Sum7 : Sum  Inputs=|++
  Sum8 : Sum  Inputs=|+-
  Switch : Switch  Criteria=u2 > Threshold
  d0 : Constant  Value=d0
  d0Lc : Constant  Value=d0Lc
  h : Constant  Value=h
  hFilterGain : Gain  Gain=hFilterGain
  hLc : Constant  Value=hLc
  vLen : Constant  Value=lr+lf
  eh : Outport
  ev : Outport  Port=2
  "gap " : Outport  Port=3
  unsafeFlag : Outport  Port=4
  wires:
  Sum6/1 -> Compare To Constant/1
  Mux/1 -> Demux1/1, Switch/3  "min safe gap"
  Sum7/1 -> Sum6/2  "safe  gap"
  Mux1/1 -> Switch/1
  d0/1 -> Mux/2
  Integrator/1 -> Demux/1, Sum5/2
  Demux1/1 -> Product/2
  Compare To Constant/1 -> unsafeFlag/1
  Sum2/1 -> eh/1
  lcFlag/1 -> Switch/2
  xl/1 -> Sum/2
  Product/1 -> Sum7/1
  h/1 -> Mux/1
  Sum3/1 -> Sum2/2  "desired  gap"
  Sum1/1 -> Sum/1  "x (front bumber)"
  vf/1 -> Sum4/1, Product/1, Multiply/1
  Sum5/1 -> hFilterGain/1
  Switch/1 -> Sum5/1
  Demux/2 -> Sum3/2
  vLen/1 -> Sum1/1
  hLc/1 -> Mux1/1
  Demux1/2 -> Sum7/2
  Multiply/1 -> Sum3/1
  Sum/1 -> Sum6/1, "gap "/1, Sum2/1  "gap"
  xf/1 -> Sum1/2
  Demux/1 -> Multiply/2
  hFilterGain/1 -> Integrator/1
  d0Lc/1 -> Mux1/2
  Sum4/1 -> ev/1
  Integrator1/1 -> Sum4/2, Sum8/2
  Gain3/1 -> Saturation/1
  Sum8/1 -> Gain3/1
  Saturation/1 -> Integrator1/1
  vl/1 -> Sum8/1

== system full_maneuver_platoon_new_strategy/Fd/Virtual Vehicle Following/Velocity Control ==
  note: Velocity control
  intReset : Inport
  ev : Inport  Port=2
  Integrator2 : Integrator  ExternalReset=rising
  Sum3 : Sum
  velKi : Gain  Gain=velKi
  velKp : Gain  Gain=velKp
  Out1 : Outport
  wires:
  Integrator2/1 -> velKi/1
  velKi/1 -> Sum3/2
  Sum3/1 -> Out1/1
  velKp/1 -> Sum3/1
  ev/1 -> velKp/1, Integrator2/1
  intReset/1 -> Integrator2/2

== system full_maneuver_platoon_new_strategy/Fd/Virtual Vehicle Following/Virtual Leader Following ==
  eh : Inport
  ev : Inport  Port=2
  realInput : Inport  Port=3
  Anti-windup gain : Gain  Gain=sqrt(Ki/Kd)
  Integrator : Integrator
  Kd : Gain  Gain=Kd
  Ki : Gain  Gain=Ki
  Kp : Gain  Gain=Kp
  Saturation1 : Saturate  UpperLimit=maxHeadwayError  LowerLimit=minHeadwayError
  Scope : Scope  NumInputPorts=4
  Sum : Sum  Inputs=|-+
  Sum1 : Sum  Inputs=+++
  Sum5 : Sum  Inputs=-+|
  u : Outport
  wires:
  ev/1 -> Kd/1
  Ki/1 -> Sum5/2
  Anti-windup gain/1 -> Sum5/1
  Sum5/1 -> Integrator/1
  Integrator/1 -> Scope/1, Sum1/1
  Kp/1 -> Scope/2, Sum1/2
  Kd/1 -> Scope/3, Sum1/3
  Saturation1/1 -> Kp/1, Ki/1
  eh/1 -> Saturation1/1
  Sum1/1 -> Scope/4, Sum/2, u/1
  realInput/1 -> Sum/1
  Sum/1 -> Anti-windup gain/1

== system full_maneuver_platoon_new_strategy/Fd/followerErrors/gapToFollower ==
  xf : Inport
  vf : Inport  Port=2
  xl : Inport  Port=3
  Multiply : Product
  Sum : Sum  Inputs=-+|
  Sum1 : Sum  Inputs=++|
  Sum2 : Sum  Inputs=+-|
  Sum3 : Sum  Inputs=|++
  d0 : Constant  Value=d0
  h : Constant  Value=h
  vLen : Constant  Value=lr+lf
  eh : Outport
  "gap " : Outport  Port=2
  wires:
  vLen/1 -> Sum1/1
  Multiply/1 -> Sum3/1
  Sum/1 -> "gap "/1, Sum2/1  "gap"
  xf/1 -> Sum1/2
  Sum3/1 -> Sum2/2  "desired  gap"
  vf/1 -> Multiply/1
  Sum1/1 -> Sum/1  "x (front bumber)"
  xl/1 -> Sum/2
  Sum2/1 -> eh/1
  h/1 -> Multiply/2  "time headway"
  d0/1 -> Sum3/2  "gap at  standstill"

== system full_maneuver_platoon_new_strategy/Fo/Lateral Control/Full State Observer ==
  note: yhat
  note: xhat
  measuredOutputs : Inport
  delta : Inport  Port=2
  Add1 : Sum  Inputs=|-+
  Gain : Gain  Gain=B  Multiplication=Matrix(K*u)
  Gain1 : Gain  Gain=C  Multiplication=Matrix(K*u)
  Gain2 : Gain  Gain=L  Multiplication=Matrix(K*u)
  Gain3 : Gain  Gain=A  Multiplication=Matrix(K*u)
  Integrator : Integrator  InitialCondition=[y0; 0; 0; 0]
  Signal Specification : SignalSpecification  Dimensions=[size(C,1) 1]
  Sum : Sum  Inputs=+++
  xhat : Outport
  wires:
  Gain2/1 -> Sum/1
  Signal Specification/1 -> Gain2/1
  Gain3/1 -> Sum/2
  Gain/1 -> Sum/3
  delta/1 -> Gain/1
  measuredOutputs/1 -> Add1/2
  Sum/1 -> Integrator/1
  Gain1/1 -> Add1/1
  Integrator/1 -> Gain1/1, Gain3/1, xhat/1
  Add1/1 -> Signal Specification/1

== system full_maneuver_platoon_new_strategy/Fo/Lateral Control/Triggered Subsystem1 ==
  In1 : Inport
  Trigger : TriggerPort  VariantControl=Variant
  Out1 : Outport  InitialOutput=y0
  wires:
  In1/1 -> Out1/1

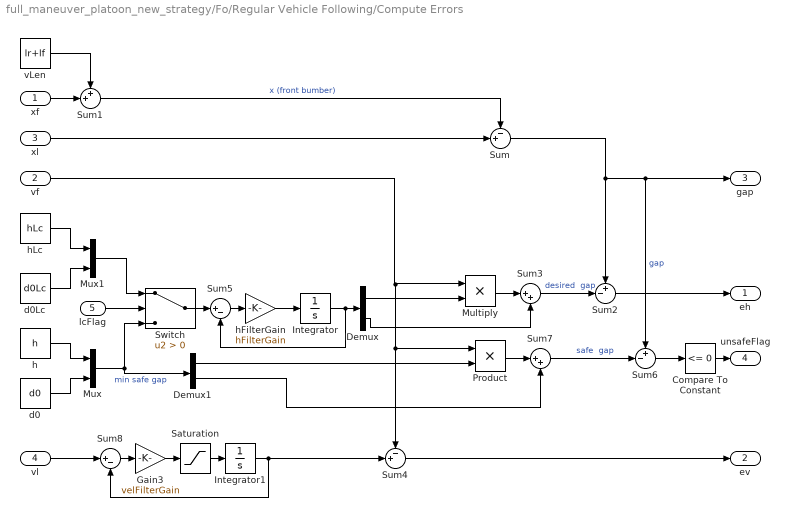
== system full_maneuver_platoon_new_strategy/Fo/Regular Vehicle Following/Compute Errors ==
  xf : Inport
  vf : Inport  Port=2
  xl : Inport  Port=3
  vl : Inport  Port=4
  lcFlag : Inport  Port=5
  Compare To Constant : simulink/Logic and Bit Operations/Compare To Constant  relop=<=  const=0  OutDataTypeStr=boolean
  Demux : Demux  Outputs=2
  Demux1 : Demux  Outputs=2
  Gain3 : Gain  Gain=velFilterGain
  Integrator : Integrator  InitialCondition=[h d0]
  Integrator1 : Integrator  InitialCondition=vx0
  Multiply : Product
  Mux : Mux  Inputs=2
  Mux1 : Mux  Inputs=2
  Product : Product
  Saturation : Saturate  UpperLimit=maxAcceleration  LowerLimit=minAcceleration
  Sum : Sum  Inputs=-+|
  Sum1 : Sum  Inputs=++|
  Sum2 : Sum  Inputs=+-|
  Sum3 : Sum  Inputs=|++
  Sum4 : Sum  Inputs=-+|
  Sum5 : Sum  Inputs=|+-
  Sum6 : Sum  Inputs=+-|
  Sum7 : Sum  Inputs=|++
  Sum8 : Sum  Inputs=|+-
  Switch : Switch  Criteria=u2 > Threshold
  d0 : Constant  Value=d0
  d0Lc : Constant  Value=d0Lc
  h : Constant  Value=h
  hFilterGain : Gain  Gain=hFilterGain
  hLc : Constant  Value=hLc
  vLen : Constant  Value=lr+lf
  eh : Outport
  ev : Outport  Port=2
  "gap " : Outport  Port=3
  unsafeFlag : Outport  Port=4
  wires:
  Sum6/1 -> Compare To Constant/1
  Mux/1 -> Demux1/1, Switch/3  "min safe gap"
  Sum7/1 -> Sum6/2  "safe  gap"
  Mux1/1 -> Switch/1
  d0/1 -> Mux/2
  Integrator/1 -> Demux/1, Sum5/2
  Demux1/1 -> Product/2
  Compare To Constant/1 -> unsafeFlag/1
  Sum2/1 -> eh/1
  lcFlag/1 -> Switch/2
  xl/1 -> Sum/2
  Product/1 -> Sum7/1
  h/1 -> Mux/1
  Sum3/1 -> Sum2/2  "desired  gap"
  Sum1/1 -> Sum/1  "x (front bumber)"
  vf/1 -> Sum4/1, Product/1, Multiply/1
  Sum5/1 -> hFilterGain/1
  Switch/1 -> Sum5/1
  Demux/2 -> Sum3/2
  vLen/1 -> Sum1/1
  hLc/1 -> Mux1/1
  Demux1/2 -> Sum7/2
  Multiply/1 -> Sum3/1
  Sum/1 -> Sum6/1, "gap "/1, Sum2/1  "gap"
  xf/1 -> Sum1/2
  Demux/1 -> Multiply/2
  hFilterGain/1 -> Integrator/1
  d0Lc/1 -> Mux1/2
  vl/1 -> Sum8/1
  Sum4/1 -> ev/1
  Gain3/1 -> Saturation/1
  Saturation/1 -> Integrator1/1
  Integrator1/1 -> Sum4/2, Sum8/2
  Sum8/1 -> Gain3/1

== system full_maneuver_platoon_new_strategy/Fo/Regular Vehicle Following/Veh Following ==
  eh : Inport
  ev : Inport  Port=2
  realInput : Inport  Port=3
  intReset : Inport  Port=4
  Anti-windup gain : Gain  Gain=sqrt(Ki/Kd)
  Integrator : Integrator  ExternalReset=rising
  Kd : Gain  Gain=Kd
  Ki : Gain  Gain=Ki
  Kp : Gain  Gain=Kp
  Saturation1 : Saturate  UpperLimit=maxHeadwayError  LowerLimit=minHeadwayError
  Scope : Scope  NumInputPorts=4
  Sum : Sum  Inputs=|-+
  Sum1 : Sum  Inputs=+++
  Sum5 : Sum  Inputs=-+|
  u : Outport
  wires:
  ev/1 -> Kd/1
  Ki/1 -> Sum5/2
  Anti-windup gain/1 -> Sum5/1
  Sum5/1 -> Integrator/1
  Integrator/1 -> Sum1/1, Scope/1
  Kp/1 -> Sum1/2, Scope/2
  Kd/1 -> Scope/3, Sum1/3
  Saturation1/1 -> Kp/1, Ki/1
  eh/1 -> Saturation1/1
  Sum1/1 -> Sum/2, u/1, Scope/4
  realInput/1 -> Sum/1
  Sum/1 -> Anti-windup gain/1
  intReset/1 -> Integrator/2
